simulink model "Design"  (R2023b)
settings: Solver=VariableStepAuto  StartTime=0.0  StopTime=10.0  RelTol=1e-3
libraries: cstblocks x8
settings Model: Creator=haita  LastModifiedBy=Albertlakers
settings RTWCC: GPUComputeCapability=5.0

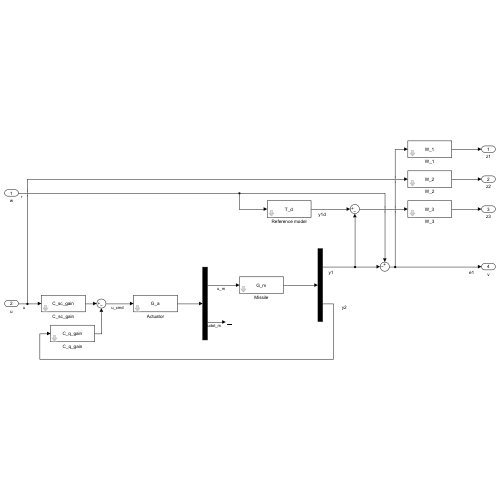
[thumbnail: Simulink's stored preview of the top-level diagram]
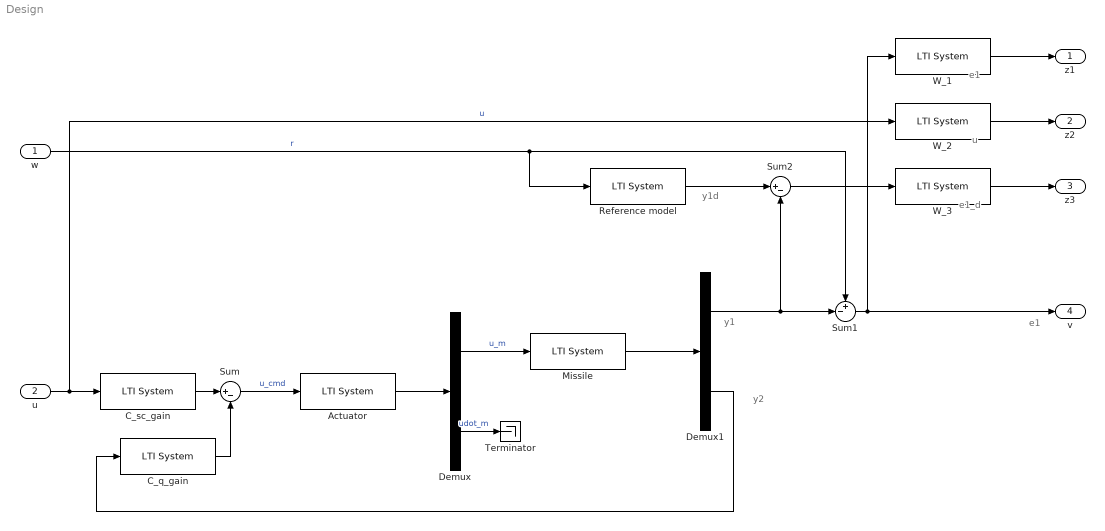
== system Design ==
  note: e1
  note: y2
  note: e1
  note: u
  note: e1_d
  note: y1
  note: y1d
  w : Inport
  u : Inport  Port=2
  Actuator : cstblocks/LTI System  sys=G_a  IC=[]  PadeOrder=0
  C_q_gain : cstblocks/LTI System  sys=C_q_gain  IC=[]  PadeOrder=0
  C_sc_gain : cstblocks/LTI System  sys=C_sc_gain  IC=[]  PadeOrder=0
  Demux : Demux  Outputs=2
  Demux1 : Demux  Outputs=2
  Missile : cstblocks/LTI System  sys=G_m  IC=[]  PadeOrder=0
  Reference model : cstblocks/LTI System  sys=T_d  IC=[]  PadeOrder=0
  Sum : Sum  Inputs=|+-
  Sum1 : Sum  Inputs=+-|
  Sum2 : Sum  Inputs=|+-
  Terminator : Terminator
  W_1 : cstblocks/LTI System  sys=W_1  IC=[]  PadeOrder=0
  W_2 : cstblocks/LTI System  sys=W_2  IC=[]  PadeOrder=0
  W_3 : cstblocks/LTI System  sys=W_3  IC=[]  PadeOrder=0
  z1 : Outport
  z2 : Outport  Port=2
  z3 : Outport  Port=3
  v : Outport  Port=4
  wires:
  Demux/1 -> Missile/1  "u_m"
  Demux/2 -> Terminator/1  "udot_m"
  Actuator/1 -> Demux/1
  u/1 -> W_2/1, C_sc_gain/1  "u"
  Demux1/2 -> C_q_gain/1
  Missile/1 -> Demux1/1
  C_q_gain/1 -> Sum/2
  Sum/1 -> Actuator/1  "u_cmd"
  C_sc_gain/1 -> Sum/1
  W_1/1 -> z1/1
  W_2/1 -> z2/1
  Demux1/1 -> Sum2/2, Sum1/2
  Sum1/1 -> W_1/1, v/1
  Reference model/1 -> Sum2/1
  Sum2/1 -> W_3/1
  w/1 -> Reference model/1, Sum1/1  "r"
  W_3/1 -> z3/1
